simulink model "UAM_GCS"  (R2024b)
settings: Solver=FixedStepAuto  StartTime=0.0  StopTime=10.0  RelTol=1e-3
undefined symbols (not defined in the file): CityMission, FixedWingMission, HoverMission, params, position, TransitionMission
settings Model: DataDictionary=UAM_data.sldd  Creator=USER  LastModifiedBy=admin
settings OptimizationCC: DefaultParameterBehavior=Inlined  EnhancedBackFolding=on  PassReuseOutputArgsAs=Individual arguments  ZeroExternalMemoryAtStartup=off  ZeroInternalMemoryAtStartup=off  OptimizeBlockOrder=speed  DifferentSizesBufferReuse=on  OptimizationCustomize=off  EfficientTunableParamExpr=on
settings DebuggingCC: ParameterTunabilityLossMsg=error
settings HardwareCC: ProdBitPerLong=64  ProdLargestAtomicInteger=LongLong  ProdLargestAtomicFloat=Double  ProdLongLongMode=on  ProdHWDeviceType=ARM Compatible->ARM Cortex-A (64-bit)
settings SFSimCC: MATLABDynamicMemAlloc=off
settings RTWCC: Description=Embedded Coder  SystemTargetFile=ert.tlc  TemplateMakefile=ert_default_tmf  Toolchain=Linaro AArch64 Linux v6.3.1
settings CodeAppCC: ForceParamTrailComments=on  IgnoreCustomStorageClasses=off  OperatorAnnotations=on  SimulinkDataObjDesc=on  SFDataObjDesc=on  CustomSymbolStrGlobalVar=GCS_$N$M  CustomSymbolStrType=GCS_$N$M_T  CustomSymbolStrField=GCS_$N$M  CustomSymbolStrFcn=GCS_$N$M$F  CustomSymbolStrBlkIO=GCS_rtb_$N$M  CustomSymbolStrTmpVar=GCS_tmp_$N$M  CustomSymbolStrMacro=GCS_$N$M_MACRO  InsertBlockDesc=on
settings ERTTargetCC: TargetLangStandard=C99 (ISO)  GenerateSampleERTMain=on  ERTCustomFileTemplate=example_file_process.tlc

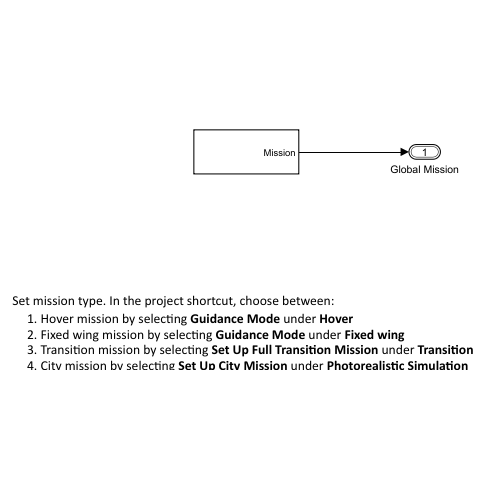
[thumbnail: Simulink's stored preview of the top-level diagram]
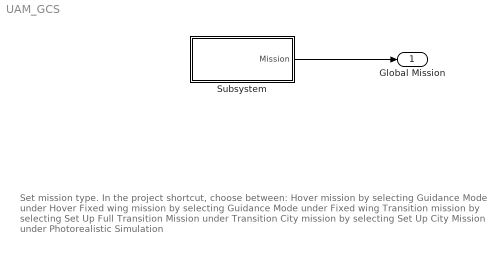
== system UAM_GCS ==
  note: Set mission type. In the project shortcut, choose between:
      | Hover mission by selecting Guidance Mode under Hover
      | Fixed wing mission by selecting Guidance Mode under Fixed wing
      | Transition mission by selecting Set Up Full Transition Mission under Transition
      | City mission by selecting Set Up City Mission under Photorealistic Simulation
  Subsystem : Subsystem
  Global Mission : Outport  OutDataTypeStr=Bus: UAVPathManagerBus  SampleTime=0.005  BusOutputAsStruct=on
  wires:
  Subsystem/1(Mission) -> Global Mission/1

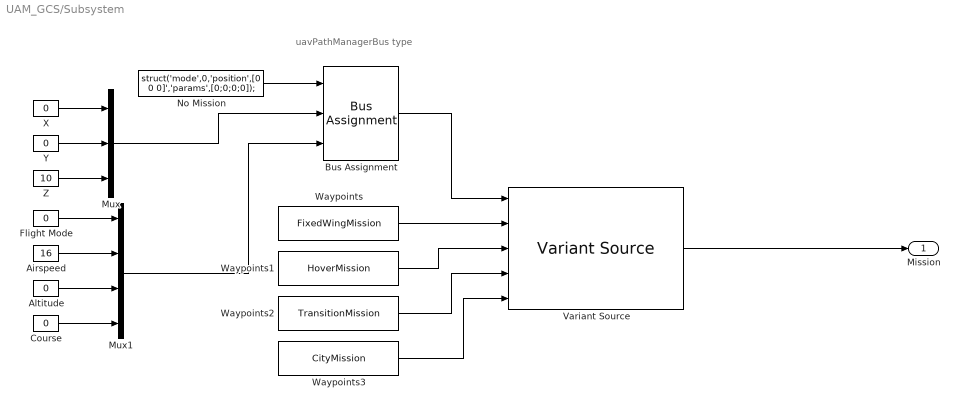
== system UAM_GCS/Subsystem ==
  note: uavPathManagerBus type
  Airspeed : Constant  Value=16
  Altitude : Constant  Value=0
  Bus Assignment : BusAssignment  AssignedSignals=position,params
  Course : Constant  Value=0
  Flight Mode : Constant  Value=0
  Mux : Mux  Inputs=3
  Mux1 : Mux
  No Mission : Constant  Value=struct('mode',0,'position',[0 0 0]','params',[0;0;0;0]);  OutDataTypeStr=Bus: UAVPathManagerBus
  Variant Source : VariantSource  ShowConditionOnBlock=on
  Waypoints : Constant  Value=FixedWingMission  OutDataTypeStr=Bus: UAVPathManagerBus  SampleTime=-1
  Waypoints1 : Constant  Value=HoverMission  OutDataTypeStr=Bus: UAVPathManagerBus  SampleTime=-1
  Waypoints2 : Constant  Value=TransitionMission  OutDataTypeStr=Bus: UAVPathManagerBus  SampleTime=-1
  Waypoints3 : Constant  Value=CityMission  OutDataTypeStr=Bus: UAVPathManagerBus  SampleTime=-1
  X : Constant  Value=0
  Y : Constant  Value=0
  Z : Constant  Value=10
  Mission : Outport
  wires:
  Waypoints1/1 -> Variant Source/3
  Airspeed/1 -> Mux1/2
  Y/1 -> Mux/2
  No Mission/1 -> Bus Assignment/1
  Z/1 -> Mux/3
  Bus Assignment/1 -> Variant Source/1
  Waypoints/1 -> Variant Source/2
  Flight Mode/1 -> Mux1/1
  X/1 -> Mux/1
  Course/1 -> Mux1/4
  Waypoints3/1 -> Variant Source/5
  Mux/1 -> Bus Assignment/2
  Waypoints2/1 -> Variant Source/4
  Altitude/1 -> Mux1/3
  Mux1/1 -> Bus Assignment/3
  Variant Source/1 -> Mission/1
